simulink model "SchemaControlloDecentralizzatoSmartSixR2010aSenzaVrep"  (Simulink 8.1)
settings: Solver=ode1  StartTime=0.0  StopTime=Tf  FixedStep=T  MaxStep=T  RelTol=1e-3
values from neighbouring files (symbols this model uses):
  Kr = diag(kr)    [MotorParametersBushelessLafert.m]
  T = 0.01    [MAIN_InitScript.m]    (also in MotorParametersBushelessLafert.m = 0.001)
CloseFcn:
  | rtwprivate ssgencode ModelCloseRequest ContributiCoppieComau
settings Model: Creator=Alessandro  LastModifiedBy=alessandromarino  ExtModeAutoUpdateStatusClock=off
settings OptimizationCC: InitFltsAndDblsToZero=on
settings DebuggingCC: SaveWithParameterizedLinksMsg=none  SignalResolutionControl=TryResolveAllWithWarning  InheritedTsInSrcMsg=none  DiscreteInheritContinuousMsg=none  MultiTaskDSMMsg=warning  MultiTaskCondExecSysMsg=none  TasksWithSamePriorityMsg=none  StrictBusMsg=None
settings GRTTargetCC: TargetFcnLib=ansi_tfl_tmw.mat

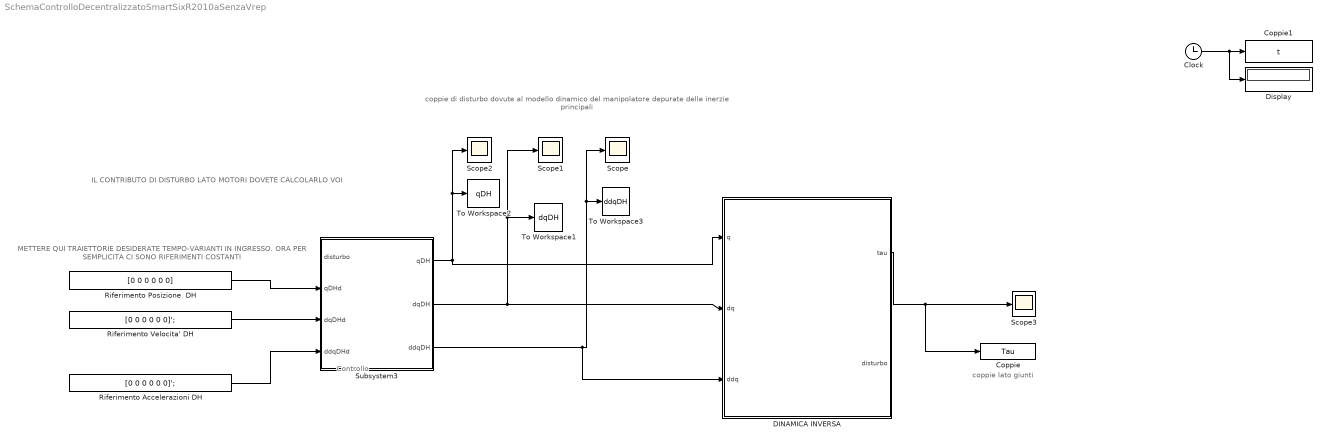
== system SchemaControlloDecentralizzatoSmartSixR2010aSenzaVrep ==
  note: coppie di disturbo dovute al modello dinamico del manipolatore depurate delle inerzie principali
  note: Controllo
  note: METTERE QUI TRAIETTORIE DESIDERATE TEMPO-VARIANTI IN INGRESSO.
      | ORA PER SEMPLICITA CI SONO RIFERIMENTI COSTANTI
  note: coppie lato giunti
  note: IL CONTRIBUTO DI DISTURBO LATO MOTORI DOVETE CALCOLARLO VOI
  Clock : Clock
  Coppie : ToWorkspace  VariableName=Tau  SampleTime=-1
  Coppie1 : ToWorkspace  VariableName=t  SampleTime=-1
  DINAMICA INVERSA : Subsystem
      mask Display:
      | disp('Contributi Coppie');
      | port_label('input', 1, 'qDH');
      | port_label('input', 2, 'dqDH');
      | port_label('input', 3, 'ddqDH');
      | port_label('output', 1, 'Coppie Complessive');
      | port_label('output', 2, 'Disturbo lato motori');
  Display : Display
  Riferimento Accelerazioni DH : Constant  Value=[0 0 0 0 0 0]';
  Riferimento Posizione  DH : Constant  Value=[0 0 0 0 0 0]
  Riferimento Velocita' DH : Constant  Value=[0 0 0 0 0 0]';
  Scope{,1..3} (4 alike) : Scope
      Scope settings: TimeRange=0.4  YMin=-300  YMax=300
      Scope1 settings: YMin=-2.75  YMax=1.25
      Scope2 settings: TimeRange=0.01894736842105263  YMin=-2  YMax=1.75  SaveName=ScopeData2
      Scope3 settings: TimeRange=0.4  YMin=-10  YMax=120  SaveName=ScopeData4
  Subsystem3 : Subsystem
      mask Display:
      | disp('Controllo');
      | port_label('input', 1, 'disturbo');
      | port_label('input', 2, 'qDHd');
      | port_label('input', 3, 'dqDHd');
      | port_label('output', 1, 'qDH');
      | port_label('output', 2, 'dqDH');
      | port_label('output', 3, 'ddqDH');
  To Workspace1 : ToWorkspace  VariableName=dqDH  SampleTime=-1
  To Workspace2 : ToWorkspace  VariableName=qDH  SampleTime=-1
  To Workspace3 : ToWorkspace  VariableName=ddqDH  SampleTime=-1
  wires:
  Clock/1 -> Coppie1/1, Display/1
  Subsystem3/2(dqDH) -> To Workspace1/1, Scope1/1, DINAMICA INVERSA/2(dq)
  DINAMICA INVERSA/1(tau) -> Scope3/1, Coppie/1
  Subsystem3/1(qDH) -> To Workspace2/1, Scope2/1, DINAMICA INVERSA/1(q)
  Subsystem3/3(ddqDH) -> To Workspace3/1, Scope/1, DINAMICA INVERSA/3(ddq)
  Riferimento Velocita' DH/1 -> Subsystem3/3(dqDHd)
  Riferimento Accelerazioni DH/1 -> Subsystem3/4(ddqDHd)
  Riferimento Posizione  DH/1 -> Subsystem3/2(qDHd)

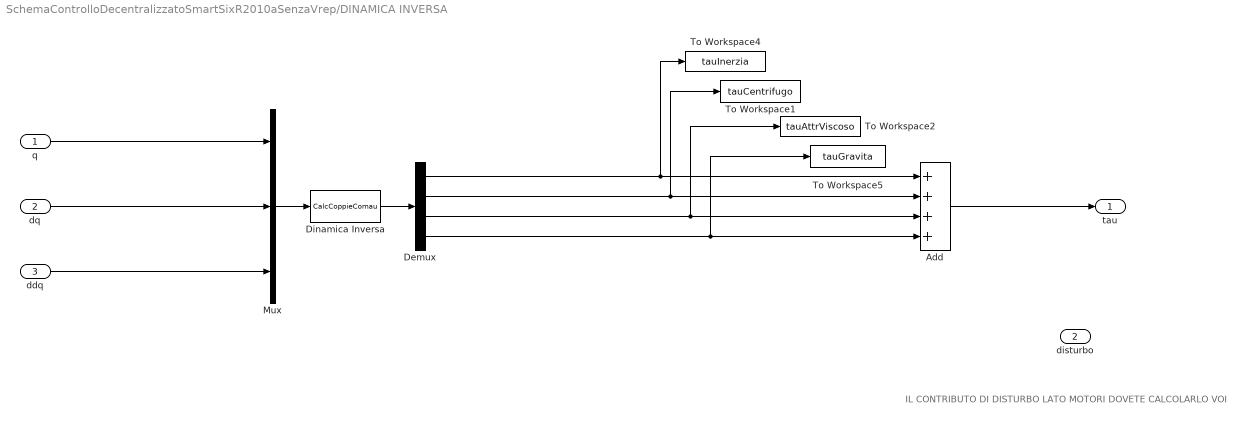
== system SchemaControlloDecentralizzatoSmartSixR2010aSenzaVrep/DINAMICA INVERSA ==
  note: IL CONTRIBUTO DI DISTURBO LATO MOTORI DOVETE CALCOLARLO VOI
  q : Inport
  dq : Inport  Port=2
  ddq : Inport  Port=3
  Add : Sum  Inputs=++++
  Demux : Demux
  Dinamica Inversa : MATLABFcn  MATLABFcn=CalcCoppieComau  OutputDimensions=24
  Mux : Mux  Inputs=3
  To Workspace1 : ToWorkspace  VariableName=tauCentrifugo  SampleTime=-1
  To Workspace2 : ToWorkspace  VariableName=tauAttrViscoso  SampleTime=-1
  To Workspace4 : ToWorkspace  VariableName=tauInerzia  SampleTime=-1
  To Workspace5 : ToWorkspace  VariableName=tauGravita  SampleTime=-1
  tau : Outport
  disturbo : Outport  Port=2
  wires:
  q/1 -> Mux/1
  Mux/1 -> Dinamica Inversa/1
  dq/1 -> Mux/2
  ddq/1 -> Mux/3
  Dinamica Inversa/1 -> Demux/1
  Add/1 -> tau/1
  Demux/1 -> Add/1, To Workspace4/1
  Demux/2 -> Add/2, To Workspace1/1
  Demux/3 -> Add/3, To Workspace2/1
  Demux/4 -> Add/4, To Workspace5/1

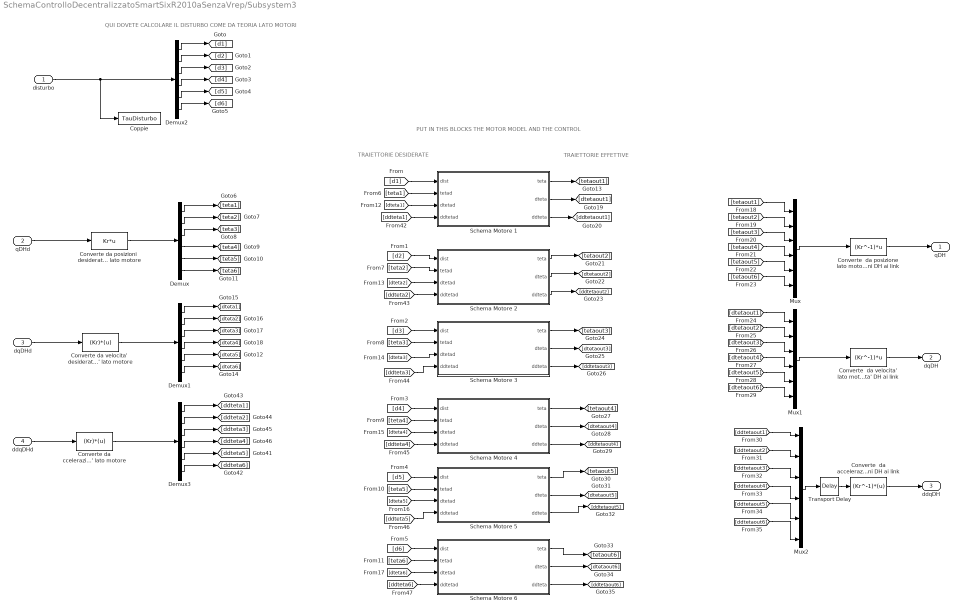
== system SchemaControlloDecentralizzatoSmartSixR2010aSenzaVrep/Subsystem3 ==
  note: PUT IN THIS BLOCKS THE MOTOR MODEL AND THE CONTROL
  note: TRAIETTORIE DESIDERATE
  note: TRAIETTORIE EFFETTIVE
  note: QUI DOVETE CALCOLARE IL DISTURBO COME DA TEORIA LATO MOTORI
  disturbo : Inport
  qDHd : Inport  Port=2
  dqDHd : Inport  Port=3
  ddqDHd : Inport  Port=4
  Converte  da accelerazioni lato motore  ad accelerazioni DH ai link : MATLABFcn  MATLABFcn=(Kr^-1)*(u)
  "Converte  da posizione lato motore a  posizioni DH ai link " : MATLABFcn  MATLABFcn=(Kr^-1)*u
  "Converte  da velocita' lato motore  a velocita' DH ai link " : MATLABFcn  MATLABFcn=(Kr^-1)*u
  Converte da ccelerazioni  desiderate DH ai link  in velocita' lato motore : MATLABFcn  MATLABFcn=(Kr)*(u)
  "Converte da posizioni  desiderate DH ai link  in posizione lato motore " : MATLABFcn  MATLABFcn=Kr*u
  "Converte da velocita'  desiderate DH ai link  in velocita' lato motore " : MATLABFcn  MATLABFcn=(Kr)*(u)
  Coppie : ToWorkspace  VariableName=TauDisturbo  SampleTime=-1
  Demux{,1..3} (4 alike) : Demux  Outputs=6
  Mux : Mux  Inputs=6
  Mux1 : Mux  Inputs=6
  Mux2 : Mux  Inputs=6
  Schema Motore 1 : Subsystem  mask{i=1}
  Schema Motore 2 : Subsystem  mask{i=2}
  Schema Motore 3 : Subsystem  mask{i=3}
  Schema Motore 4 : Subsystem  mask{i=4}
  Schema Motore 5 : Subsystem  mask{i=5}
  Schema Motore 6 : Subsystem  mask{i=6}
  Transport Delay : TransportDelay  DelayTime=T
  qDH : Outport
  dqDH : Outport  Port=2
  ddqDH : Outport  Port=3
  wires:
  qDHd/1 -> "Converte da posizioni  desiderate DH ai link  in posizione lato motore "/1
  dqDHd/1 -> "Converte da velocita'  desiderate DH ai link  in velocita' lato motore "/1
  "Converte  da velocita' lato motore  a velocita' DH ai link "/1 -> dqDH/1
  Converte  da accelerazioni lato motore  ad accelerazioni DH ai link/1 -> ddqDH/1
  "Converte da posizioni  desiderate DH ai link  in posizione lato motore "/1 -> Demux/1
  disturbo/1 -> Coppie/1, Demux2/1
  "Converte  da posizione lato motore a  posizioni DH ai link "/1 -> qDH/1
  Mux/1 -> "Converte  da posizione lato motore a  posizioni DH ai link "/1
  Demux2/1 -> [d1]
  Demux2/2 -> [d2]
  Demux2/3 -> [d3]
  Demux2/4 -> [d4]
  Demux2/5 -> [d5]
  Demux2/6 -> [d6]
  [d3] -> Schema Motore 3/1(dist)
  [d4] -> Schema Motore 4/1(dist)
  [d5] -> Schema Motore 5/1(dist)
  [d6] -> Schema Motore 6/1(dist)
  Demux/1 -> [teta1]
  Demux/2 -> [teta2]
  Demux/3 -> [teta3]
  Demux/4 -> [teta4]
  Demux/5 -> [teta5]
  Demux/6 -> [teta6]
  [teta2] -> Schema Motore 2/2(tetad)
  [teta3] -> Schema Motore 3/2(tetad)
  [teta4] -> Schema Motore 4/2(tetad)
  [teta5] -> Schema Motore 5/2(tetad)
  [teta6] -> Schema Motore 6/2(tetad)
  "Converte da velocita'  desiderate DH ai link  in velocita' lato motore "/1 -> Demux1/1
  Demux1/1 -> [dteta1]
  Demux1/2 -> [dteta2]
  Demux1/3 -> [dteta3]
  Demux1/4 -> [dteta4]
  Demux1/5 -> [dteta5]
  Demux1/6 -> [dteta6]
  [dteta2] -> Schema Motore 2/3(dtetad)
  [dteta3] -> Schema Motore 3/3(dtetad)
  [dteta4] -> Schema Motore 4/3(dtetad)
  [dteta5] -> Schema Motore 5/3(dtetad)
  [dteta6] -> Schema Motore 6/3(dtetad)
  [tetaout1] -> Mux/1
  [tetaout2] -> Mux/2
  [tetaout3] -> Mux/3
  [tetaout4] -> Mux/4
  [tetaout5] -> Mux/5
  [tetaout6] -> Mux/6
  Mux1/1 -> "Converte  da velocita' lato motore  a velocita' DH ai link "/1
  [dtetaout1] -> Mux1/1
  [dtetaout2] -> Mux1/2
  [dtetaout3] -> Mux1/3
  [dtetaout4] -> Mux1/4
  [dtetaout5] -> Mux1/5
  [dtetaout6] -> Mux1/6
  Mux2/1 -> Transport Delay/1
  [ddtetaout1] -> Mux2/1
  [ddtetaout2] -> Mux2/2
  [ddtetaout3] -> Mux2/3
  [ddtetaout4] -> Mux2/4
  [ddtetaout5] -> Mux2/5
  [ddtetaout6] -> Mux2/6
  Schema Motore 2/1(teta) -> [tetaout2]
  Schema Motore 2/2(dteta) -> [dtetaout2]
  Schema Motore 2/3(ddteta) -> [ddtetaout2]
  Transport Delay/1 -> Converte  da accelerazioni lato motore  ad accelerazioni DH ai link/1
  [d2] -> Schema Motore 2/1(dist)
  [teta1] -> Schema Motore 1/2(tetad)
  [dteta1] -> Schema Motore 1/3(dtetad)
  Schema Motore 1/1(teta) -> [tetaout1]
  Schema Motore 1/2(dteta) -> [dtetaout1]
  Schema Motore 1/3(ddteta) -> [ddtetaout1]
  [d1] -> Schema Motore 1/1(dist)
  ddqDHd/1 -> Converte da ccelerazioni  desiderate DH ai link  in velocita' lato motore/1
  Demux3/1 -> [ddteta1]
  Demux3/2 -> [ddteta2]
  Demux3/3 -> [ddteta3]
  Demux3/4 -> [ddteta4]
  Demux3/5 -> [ddteta5]
  Demux3/6 -> [ddteta6]
  Converte da ccelerazioni  desiderate DH ai link  in velocita' lato motore/1 -> Demux3/1
  [ddteta1] -> Schema Motore 1/4(ddtetad)
  Schema Motore 3/1(teta) -> [tetaout3]
  Schema Motore 3/2(dteta) -> [dtetaout3]
  Schema Motore 3/3(ddteta) -> [ddtetaout3]
  Schema Motore 4/1(teta) -> [tetaout4]
  Schema Motore 4/2(dteta) -> [dtetaout4]
  Schema Motore 4/3(ddteta) -> [ddtetaout4]
  Schema Motore 5/1(teta) -> [tetaout5]
  Schema Motore 5/2(dteta) -> [dtetaout5]
  Schema Motore 5/3(ddteta) -> [ddtetaout5]
  Schema Motore 6/1(teta) -> [tetaout6]
  Schema Motore 6/2(dteta) -> [dtetaout6]
  Schema Motore 6/3(ddteta) -> [ddtetaout6]
  [ddteta2] -> Schema Motore 2/4(ddtetad)
  [ddteta3] -> Schema Motore 3/4(ddtetad)
  [ddteta4] -> Schema Motore 4/4(ddtetad)
  [ddteta5] -> Schema Motore 5/4(ddtetad)
  [ddteta6] -> Schema Motore 6/4(ddtetad)

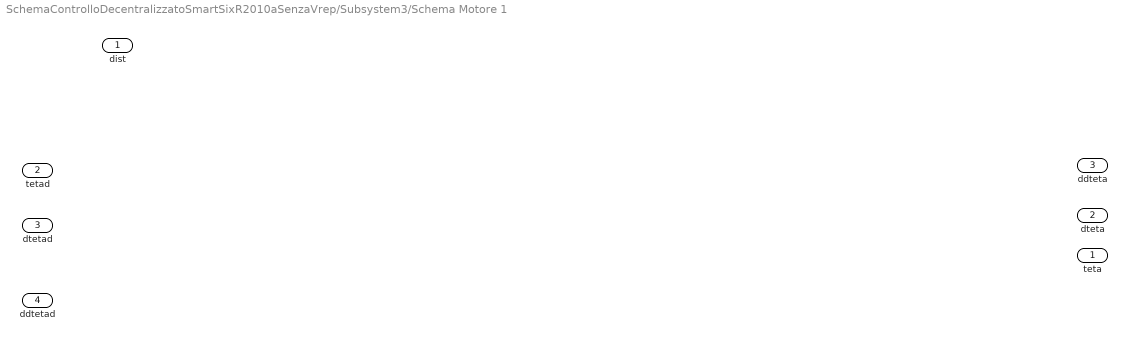
== system SchemaControlloDecentralizzatoSmartSixR2010aSenzaVrep/Subsystem3/Schema Motore 1 ==
  dist : Inport  PortDimensions=1
  tetad : Inport  Port=2  PortDimensions=1
  dtetad : Inport  Port=3  PortDimensions=1
  ddtetad : Inport  Port=4  PortDimensions=1
  teta : Outport  PortDimensions=1
  dteta : Outport  Port=2  PortDimensions=1
  ddteta : Outport  Port=3  PortDimensions=1

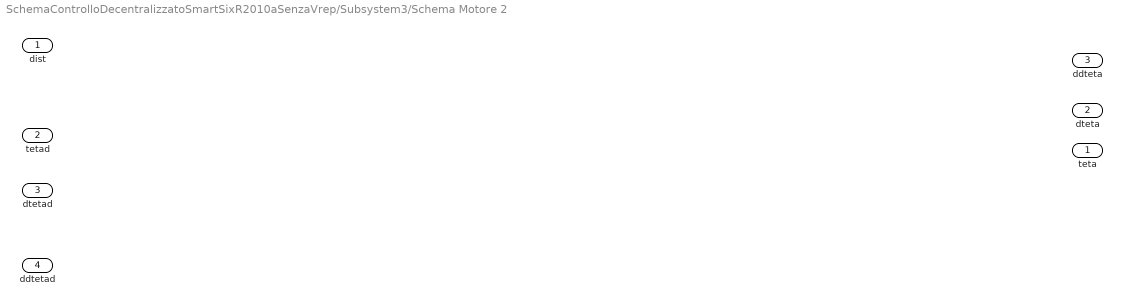
== system SchemaControlloDecentralizzatoSmartSixR2010aSenzaVrep/Subsystem3/Schema Motore 2 ==
  dist : Inport  PortDimensions=1
  tetad : Inport  Port=2  PortDimensions=1
  dtetad : Inport  Port=3  PortDimensions=1
  ddtetad : Inport  Port=4  PortDimensions=1
  teta : Outport  PortDimensions=1
  dteta : Outport  Port=2  PortDimensions=1
  ddteta : Outport  Port=3  PortDimensions=1

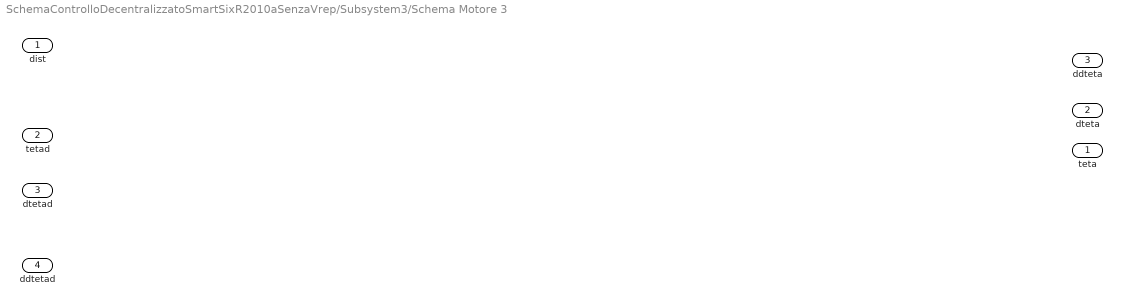
== system SchemaControlloDecentralizzatoSmartSixR2010aSenzaVrep/Subsystem3/Schema Motore 3 ==
  dist : Inport  PortDimensions=1
  tetad : Inport  Port=2  PortDimensions=1
  dtetad : Inport  Port=3  PortDimensions=1
  ddtetad : Inport  Port=4  PortDimensions=1
  teta : Outport  PortDimensions=1
  dteta : Outport  Port=2  PortDimensions=1
  ddteta : Outport  Port=3  PortDimensions=1

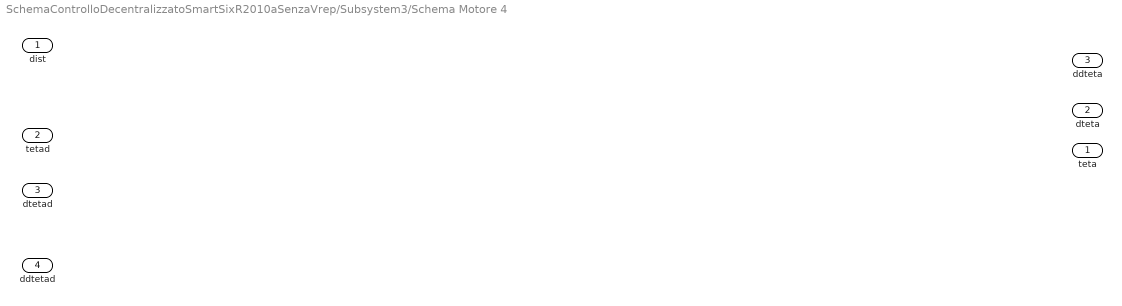
== system SchemaControlloDecentralizzatoSmartSixR2010aSenzaVrep/Subsystem3/Schema Motore 4 ==
  dist : Inport  PortDimensions=1
  tetad : Inport  Port=2  PortDimensions=1
  dtetad : Inport  Port=3  PortDimensions=1
  ddtetad : Inport  Port=4  PortDimensions=1
  teta : Outport  PortDimensions=1
  dteta : Outport  Port=2  PortDimensions=1
  ddteta : Outport  Port=3  PortDimensions=1

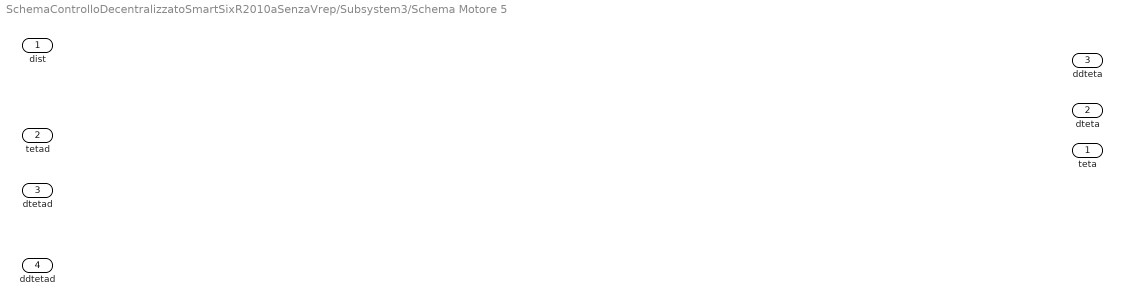
== system SchemaControlloDecentralizzatoSmartSixR2010aSenzaVrep/Subsystem3/Schema Motore 5 ==
  dist : Inport  PortDimensions=1
  tetad : Inport  Port=2  PortDimensions=1
  dtetad : Inport  Port=3  PortDimensions=1
  ddtetad : Inport  Port=4  PortDimensions=1
  teta : Outport  PortDimensions=1
  dteta : Outport  Port=2  PortDimensions=1
  ddteta : Outport  Port=3  PortDimensions=1

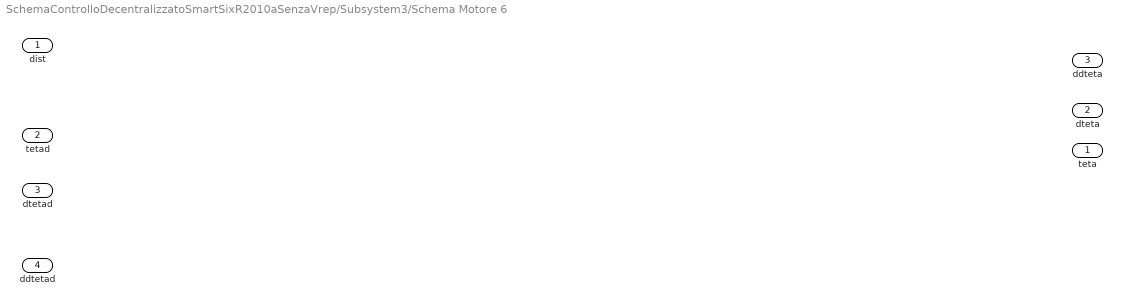
== system SchemaControlloDecentralizzatoSmartSixR2010aSenzaVrep/Subsystem3/Schema Motore 6 ==
  dist : Inport  PortDimensions=1
  tetad : Inport  Port=2  PortDimensions=1
  dtetad : Inport  Port=3  PortDimensions=1
  ddtetad : Inport  Port=4  PortDimensions=1
  teta : Outport  PortDimensions=1
  dteta : Outport  Port=2  PortDimensions=1
  ddteta : Outport  Port=3  PortDimensions=1
